simulink library "MotionFilter_Library"  (R2025a)
settings: Solver=VariableStepAuto  StartTime=0.0  StopTime=10.0  RelTol=1e-3
settings Model: Creator=damerius  LastModifiedBy=damerius

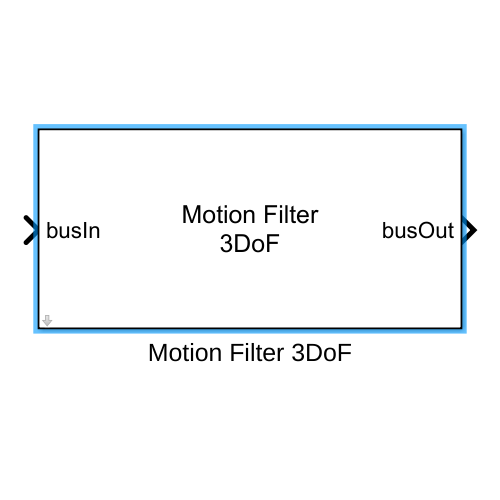
[thumbnail: Simulink's stored preview of the top-level diagram]
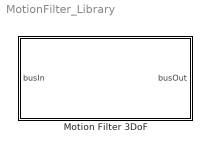
== system MotionFilter_Library ==
  Motion Filter 3DoF : Subsystem
      mask help:
      | Motion filter for a surface vehicle that estimates pose and velocity as well as an external force acting on the vehicle. This block provides a simulink interface for the MotionFilter3DoF class. For more information on this filter, run '<i>help motionfilter.MotionFilter3DoF</i>' from the MATLAB command window.<br><br>
      | <b>busIn</b><br>Input bus of type 'busMotionFilter3DoFIn'.<br><br>
      | <b>busOut</b><br>Output bus of type 'busMotionFilter3DoFOut'.<br><br>
      mask DialogControl DescGroupVar Prompt: Motion Filter 3DoF
      mask Display: disp('Motion Filter\n3DoF');

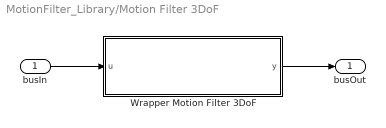
== system MotionFilter_Library/Motion Filter 3DoF ==
  busIn : Inport  OutDataTypeStr=Bus: busMotionFilter3DoFIn
  Wrapper Motion Filter 3DoF : MATLAB Function  TreatAsAtomicUnit=on
  busOut : Outport  OutDataTypeStr=Bus: busMotionFilter3DoFOut
  wires:
  busIn/1 -> Wrapper Motion Filter 3DoF/1(u)
  Wrapper Motion Filter 3DoF/1(y) -> busOut/1

== matlab function MotionFilter_Library/Motion Filter 3DoF/Wrapper Motion Filter 3DoF ==
  data: u input Bus: busMotionFilter3DoFIn; y output Bus: busMotionFilter3DoFOut
function y = Wrapper_MotionFilter3DoF(u)
    persistent motionFilter;
    if(isempty(motionFilter))
        motionFilter = motionfilter.MotionFilter3DoF();
    end
    y = motionFilter.Step(u);
end
